simulink model "three"  (R2014b)
settings: Solver=ode23tb  StartTime=0.0  StopTime=0.1  MaxStep=.0001  MinStep=0.00001  RelTol=1e-3
libraries: powerlib x120, simulink x60, powerlib_meascontrol x1
(part 2 of 2)

== system three/R/R/LOOKUP TABLE/If Action Subsystem1 ==
  In1 : Inport
  Action Port : ActionPort  ActionType=case
  Out1 : Outport
  wires:
  In1/1 -> Out1/1

== system three/R/R/LOOKUP TABLE/If Action Subsystem10 ==
  In1 : Inport
  Action Port : ActionPort  ActionType=case
  Out1 : Outport
  wires:
  In1/1 -> Out1/1

== system three/R/R/LOOKUP TABLE/If Action Subsystem2 ==
  In1 : Inport
  Action Port : ActionPort  ActionType=case
  Out1 : Outport
  wires:
  In1/1 -> Out1/1

== system three/R/R/LOOKUP TABLE/If Action Subsystem3 ==
  In1 : Inport
  Action Port : ActionPort  ActionType=case
  Out1 : Outport
  wires:
  In1/1 -> Out1/1

== system three/R/R/LOOKUP TABLE/If Action Subsystem4 ==
  In1 : Inport
  Action Port : ActionPort  ActionType=case
  Out1 : Outport
  wires:
  In1/1 -> Out1/1

== system three/R/R/LOOKUP TABLE/If Action Subsystem5 ==
  In1 : Inport
  Action Port : ActionPort  ActionType=case
  Out1 : Outport
  wires:
  In1/1 -> Out1/1

== system three/R/R/LOOKUP TABLE/If Action Subsystem6 ==
  In1 : Inport
  Action Port : ActionPort  ActionType=case
  Out1 : Outport
  wires:
  In1/1 -> Out1/1

== system three/R/R/LOOKUP TABLE/If Action Subsystem7 ==
  In1 : Inport
  Action Port : ActionPort  ActionType=case
  Out1 : Outport
  wires:
  In1/1 -> Out1/1

== system three/R/R/LOOKUP TABLE/If Action Subsystem8 ==
  In1 : Inport
  Action Port : ActionPort  ActionType=case
  Out1 : Outport
  wires:
  In1/1 -> Out1/1

== system three/R/R/LOOKUP TABLE/If Action Subsystem9 ==
  In1 : Inport
  Action Port : ActionPort  ActionType=case
  Out1 : Outport
  wires:
  In1/1 -> Out1/1

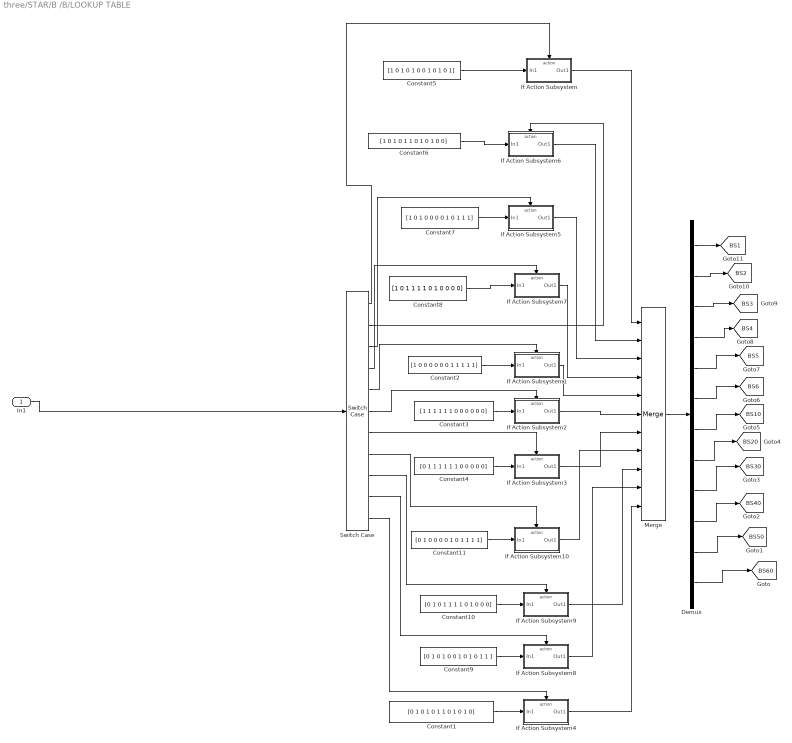
== system three/STAR/B /B/LOOKUP TABLE ==
  In1 : Inport
  Constant1 : Constant  Value=[0 1 0 1 0 1 1 0 1 0 1 0]
  Constant10 : Constant  Value=[0 1 0 1 1 1 1 0 1 0 0 0]
  Constant11 : Constant  Value=[0 1 0 0 0 0 1 0 1 1 1 1]
  Constant2 : Constant  Value=[1 0 0 0 0 0 0 1 1 1 1 1]
  Constant3 : Constant  Value=[1 1 1 1 1 1 0 0 0 0 0 0]
  Constant4 : Constant  Value=[0 1 1 1 1 1 1 0 0 0 0 0]
  Constant5 : Constant  Value=[1 0 1 0 1 0 0 1 0 1 0 1]
  Constant6 : Constant  Value=[1 0 1 0 1 1 0 1 0 1 0 0]
  Constant7 : Constant  Value=[1 0 1 0 0 0 0 1 0 1 1 1]
  Constant8 : Constant  Value=[1 0 1 1 1 1 0 1 0 0 0 0]
  Constant9 : Constant  Value=[0 1 0 1 0 0 1 0 1 0 1 1 ]
  Demux : Demux  Outputs=12
  If Action Subsystem : Subsystem  TreatAsAtomicUnit=on
  If Action Subsystem1 : Subsystem  TreatAsAtomicUnit=on
  If Action Subsystem10 : Subsystem  TreatAsAtomicUnit=on
  If Action Subsystem2 : Subsystem  TreatAsAtomicUnit=on
  If Action Subsystem3 : Subsystem  TreatAsAtomicUnit=on
  If Action Subsystem4 : Subsystem  TreatAsAtomicUnit=on
  If Action Subsystem5 : Subsystem  TreatAsAtomicUnit=on
  If Action Subsystem6 : Subsystem  TreatAsAtomicUnit=on
  If Action Subsystem7 : Subsystem  TreatAsAtomicUnit=on
  If Action Subsystem8 : Subsystem  TreatAsAtomicUnit=on
  If Action Subsystem9 : Subsystem  TreatAsAtomicUnit=on
  Merge : Merge  Inputs=11
  Switch Case : SwitchCase  CaseConditions={-5 -4 -3 -2 -1 0 1 2 3 4 5}  ShowDefaultCase=off
  tag scope: BS10=global, BS1=global, BS20=global, BS2=global, BS30=global, BS3=global, BS40=global, BS4=global, BS50=global, BS5=global, BS60=global, BS6=global
  wires:
  Merge/1 -> Demux/1
  If Action Subsystem/1(Out1) -> Merge/1
  Constant4/1 -> If Action Subsystem3/1(In1)
  Constant3/1 -> If Action Subsystem2/1(In1)
  Constant2/1 -> If Action Subsystem1/1(In1)
  Switch Case/6 -> If Action Subsystem2/Action
  If Action Subsystem6/1(Out1) -> Merge/2
  If Action Subsystem5/1(Out1) -> Merge/3
  If Action Subsystem7/1(Out1) -> Merge/4
  If Action Subsystem1/1(Out1) -> Merge/5
  If Action Subsystem2/1(Out1) -> Merge/6
  If Action Subsystem3/1(Out1) -> Merge/7
  Constant9/1 -> If Action Subsystem8/1(In1)
  Constant10/1 -> If Action Subsystem9/1(In1)
  Constant11/1 -> If Action Subsystem10/1(In1)
  Switch Case/11 -> If Action Subsystem4/Action
  If Action Subsystem4/1(Out1) -> Merge/11
  Switch Case/10 -> If Action Subsystem8/Action
  Switch Case/9 -> If Action Subsystem9/Action
  Switch Case/8 -> If Action Subsystem10/Action
  Switch Case/7 -> If Action Subsystem3/Action
  Switch Case/5 -> If Action Subsystem1/Action
  Switch Case/4 -> If Action Subsystem7/Action
  Switch Case/3 -> If Action Subsystem5/Action
  Switch Case/2 -> If Action Subsystem6/Action
  Switch Case/1 -> If Action Subsystem/Action
  Constant6/1 -> If Action Subsystem6/1(In1)
  Constant7/1 -> If Action Subsystem5/1(In1)
  Constant8/1 -> If Action Subsystem7/1(In1)
  If Action Subsystem10/1(Out1) -> Merge/8
  If Action Subsystem9/1(Out1) -> Merge/9
  If Action Subsystem8/1(Out1) -> Merge/10
  Constant1/1 -> If Action Subsystem4/1(In1)
  Constant5/1 -> If Action Subsystem/1(In1)
  In1/1 -> Switch Case/1
  Demux/1 -> [BS1]
  Demux/2 -> [BS2]
  Demux/3 -> [BS3]
  Demux/4 -> [BS4]
  Demux/6 -> [BS6]
  Demux/5 -> [BS5]
  Demux/7 -> [BS10]
  Demux/8 -> [BS20]
  Demux/11 -> [BS50]
  Demux/10 -> [BS40]
  Demux/9 -> [BS30]
  Demux/12 -> [BS60]

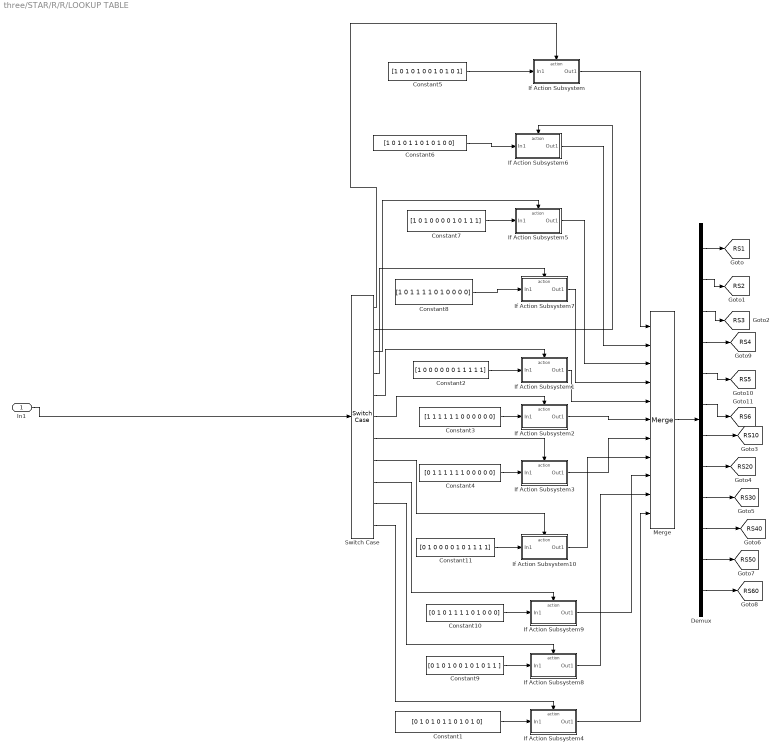
== system three/STAR/R/R/LOOKUP TABLE ==
  In1 : Inport
  Constant1 : Constant  Value=[0 1 0 1 0 1 1 0 1 0 1 0]
  Constant10 : Constant  Value=[0 1 0 1 1 1 1 0 1 0 0 0]
  Constant11 : Constant  Value=[0 1 0 0 0 0 1 0 1 1 1 1]
  Constant2 : Constant  Value=[1 0 0 0 0 0 0 1 1 1 1 1]
  Constant3 : Constant  Value=[1 1 1 1 1 1 0 0 0 0 0 0]
  Constant4 : Constant  Value=[0 1 1 1 1 1 1 0 0 0 0 0]
  Constant5 : Constant  Value=[1 0 1 0 1 0 0 1 0 1 0 1]
  Constant6 : Constant  Value=[1 0 1 0 1 1 0 1 0 1 0 0]
  Constant7 : Constant  Value=[1 0 1 0 0 0 0 1 0 1 1 1]
  Constant8 : Constant  Value=[1 0 1 1 1 1 0 1 0 0 0 0]
  Constant9 : Constant  Value=[0 1 0 1 0 0 1 0 1 0 1 1 ]
  Demux : Demux  Outputs=12
  If Action Subsystem : Subsystem  TreatAsAtomicUnit=on
  If Action Subsystem1 : Subsystem  TreatAsAtomicUnit=on
  If Action Subsystem10 : Subsystem  TreatAsAtomicUnit=on
  If Action Subsystem2 : Subsystem  TreatAsAtomicUnit=on
  If Action Subsystem3 : Subsystem  TreatAsAtomicUnit=on
  If Action Subsystem4 : Subsystem  TreatAsAtomicUnit=on
  If Action Subsystem5 : Subsystem  TreatAsAtomicUnit=on
  If Action Subsystem6 : Subsystem  TreatAsAtomicUnit=on
  If Action Subsystem7 : Subsystem  TreatAsAtomicUnit=on
  If Action Subsystem8 : Subsystem  TreatAsAtomicUnit=on
  If Action Subsystem9 : Subsystem  TreatAsAtomicUnit=on
  Merge : Merge  Inputs=11
  Switch Case : SwitchCase  CaseConditions={-5 -4 -3 -2 -1 0 1 2 3 4 5}  ShowDefaultCase=off
  tag scope: RS10=global, RS1=global, RS20=global, RS2=global, RS30=global, RS3=global, RS40=global, RS4=global, RS50=global, RS5=global, RS60=global, RS6=global
  wires:
  Merge/1 -> Demux/1
  If Action Subsystem/1(Out1) -> Merge/1
  Constant4/1 -> If Action Subsystem3/1(In1)
  Constant3/1 -> If Action Subsystem2/1(In1)
  Constant2/1 -> If Action Subsystem1/1(In1)
  Switch Case/6 -> If Action Subsystem2/Action
  If Action Subsystem6/1(Out1) -> Merge/2
  If Action Subsystem5/1(Out1) -> Merge/3
  If Action Subsystem7/1(Out1) -> Merge/4
  If Action Subsystem1/1(Out1) -> Merge/5
  If Action Subsystem2/1(Out1) -> Merge/6
  If Action Subsystem3/1(Out1) -> Merge/7
  Constant9/1 -> If Action Subsystem8/1(In1)
  Constant10/1 -> If Action Subsystem9/1(In1)
  Constant11/1 -> If Action Subsystem10/1(In1)
  Switch Case/11 -> If Action Subsystem4/Action
  If Action Subsystem4/1(Out1) -> Merge/11
  Switch Case/10 -> If Action Subsystem8/Action
  Switch Case/9 -> If Action Subsystem9/Action
  Switch Case/8 -> If Action Subsystem10/Action
  Switch Case/7 -> If Action Subsystem3/Action
  Switch Case/5 -> If Action Subsystem1/Action
  Switch Case/4 -> If Action Subsystem7/Action
  Switch Case/3 -> If Action Subsystem5/Action
  Switch Case/2 -> If Action Subsystem6/Action
  Switch Case/1 -> If Action Subsystem/Action
  Constant6/1 -> If Action Subsystem6/1(In1)
  Constant7/1 -> If Action Subsystem5/1(In1)
  Constant8/1 -> If Action Subsystem7/1(In1)
  If Action Subsystem10/1(Out1) -> Merge/8
  If Action Subsystem9/1(Out1) -> Merge/9
  If Action Subsystem8/1(Out1) -> Merge/10
  Demux/3 -> [RS3]
  Demux/2 -> [RS2]
  Demux/1 -> [RS1]
  Demux/7 -> [RS10]
  Demux/8 -> [RS20]
  Demux/9 -> [RS30]
  Demux/10 -> [RS40]
  Demux/11 -> [RS50]
  Demux/12 -> [RS60]
  Demux/6 -> [RS6]
  Demux/5 -> [RS5]
  Demux/4 -> [RS4]
  Constant1/1 -> If Action Subsystem4/1(In1)
  Constant5/1 -> If Action Subsystem/1(In1)
  In1/1 -> Switch Case/1

== system three/STAR/Y/B/LOOKUP TABLE ==
  In1 : Inport
  Constant1 : Constant  Value=[0 1 0 1 0 1 1 0 1 0 1 0]
  Constant10 : Constant  Value=[0 1 0 1 1 1 1 0 1 0 0 0]
  Constant11 : Constant  Value=[0 1 0 0 0 0 1 0 1 1 1 1]
  Constant2 : Constant  Value=[1 0 0 0 0 0 0 1 1 1 1 1]
  Constant3 : Constant  Value=[1 1 1 1 1 1 0 0 0 0 0 0]
  Constant4 : Constant  Value=[0 1 1 1 1 1 1 0 0 0 0 0]
  Constant5 : Constant  Value=[1 0 1 0 1 0 0 1 0 1 0 1]
  Constant6 : Constant  Value=[1 0 1 0 1 1 0 1 0 1 0 0]
  Constant7 : Constant  Value=[1 0 1 0 0 0 0 1 0 1 1 1]
  Constant8 : Constant  Value=[1 0 1 1 1 1 0 1 0 0 0 0]
  Constant9 : Constant  Value=[0 1 0 1 0 0 1 0 1 0 1 1 ]
  Demux : Demux  Outputs=12
  If Action Subsystem : Subsystem  TreatAsAtomicUnit=on
  If Action Subsystem1 : Subsystem  TreatAsAtomicUnit=on
  If Action Subsystem10 : Subsystem  TreatAsAtomicUnit=on
  If Action Subsystem2 : Subsystem  TreatAsAtomicUnit=on
  If Action Subsystem3 : Subsystem  TreatAsAtomicUnit=on
  If Action Subsystem4 : Subsystem  TreatAsAtomicUnit=on
  If Action Subsystem5 : Subsystem  TreatAsAtomicUnit=on
  If Action Subsystem6 : Subsystem  TreatAsAtomicUnit=on
  If Action Subsystem7 : Subsystem  TreatAsAtomicUnit=on
  If Action Subsystem8 : Subsystem  TreatAsAtomicUnit=on
  If Action Subsystem9 : Subsystem  TreatAsAtomicUnit=on
  Merge : Merge  Inputs=11
  Switch Case : SwitchCase  CaseConditions={-5 -4 -3 -2 -1 0 1 2 3 4 5}  ShowDefaultCase=off
  tag scope: YS10=global, YS20=global, YS2=global, YS30=global, YS3=global, YS40=global, YS4=global, YS50=global, YS5=global, YS60=global, YS6=global
  wires:
  In1/1 -> Switch Case/1
  Constant5/1 -> If Action Subsystem/1(In1)
  Constant1/1 -> If Action Subsystem4/1(In1)
  If Action Subsystem8/1(Out1) -> Merge/10
  If Action Subsystem9/1(Out1) -> Merge/9
  If Action Subsystem10/1(Out1) -> Merge/8
  Constant8/1 -> If Action Subsystem7/1(In1)
  Constant7/1 -> If Action Subsystem5/1(In1)
  Constant6/1 -> If Action Subsystem6/1(In1)
  Switch Case/1 -> If Action Subsystem/Action
  Switch Case/2 -> If Action Subsystem6/Action
  Switch Case/3 -> If Action Subsystem5/Action
  Switch Case/4 -> If Action Subsystem7/Action
  Switch Case/5 -> If Action Subsystem1/Action
  Switch Case/7 -> If Action Subsystem3/Action
  Switch Case/8 -> If Action Subsystem10/Action
  Switch Case/9 -> If Action Subsystem9/Action
  Switch Case/10 -> If Action Subsystem8/Action
  If Action Subsystem4/1(Out1) -> Merge/11
  Switch Case/11 -> If Action Subsystem4/Action
  Constant11/1 -> If Action Subsystem10/1(In1)
  Constant10/1 -> If Action Subsystem9/1(In1)
  Constant9/1 -> If Action Subsystem8/1(In1)
  If Action Subsystem3/1(Out1) -> Merge/7
  If Action Subsystem2/1(Out1) -> Merge/6
  If Action Subsystem1/1(Out1) -> Merge/5
  If Action Subsystem7/1(Out1) -> Merge/4
  If Action Subsystem5/1(Out1) -> Merge/3
  If Action Subsystem6/1(Out1) -> Merge/2
  Switch Case/6 -> If Action Subsystem2/Action
  Constant2/1 -> If Action Subsystem1/1(In1)
  Constant3/1 -> If Action Subsystem2/1(In1)
  Constant4/1 -> If Action Subsystem3/1(In1)
  If Action Subsystem/1(Out1) -> Merge/1
  Merge/1 -> Demux/1
  Demux/1 -> [YS1]
  Demux/3 -> [YS3]
  Demux/2 -> [YS2]
  Demux/4 -> [YS4]
  Demux/5 -> [YS5]
  Demux/6 -> [YS6]
  Demux/7 -> [YS10]
  Demux/8 -> [YS20]
  Demux/9 -> [YS30]
  Demux/10 -> [YS40]
  Demux/11 -> [YS50]
  Demux/12 -> [YS60]

== system three/Y/Y/LOOKUP TABLE/If Action Subsystem ==
  In1 : Inport
  Action Port : ActionPort  ActionType=case
  Out1 : Outport
  wires:
  In1/1 -> Out1/1

== system three/Y/Y/LOOKUP TABLE/If Action Subsystem1 ==
  In1 : Inport
  Action Port : ActionPort  ActionType=case
  Out1 : Outport
  wires:
  In1/1 -> Out1/1

== system three/Y/Y/LOOKUP TABLE/If Action Subsystem10 ==
  In1 : Inport
  Action Port : ActionPort  ActionType=case
  Out1 : Outport
  wires:
  In1/1 -> Out1/1

== system three/Y/Y/LOOKUP TABLE/If Action Subsystem2 ==
  In1 : Inport
  Action Port : ActionPort  ActionType=case
  Out1 : Outport
  wires:
  In1/1 -> Out1/1

== system three/Y/Y/LOOKUP TABLE/If Action Subsystem3 ==
  In1 : Inport
  Action Port : ActionPort  ActionType=case
  Out1 : Outport
  wires:
  In1/1 -> Out1/1

== system three/Y/Y/LOOKUP TABLE/If Action Subsystem4 ==
  In1 : Inport
  Action Port : ActionPort  ActionType=case
  Out1 : Outport
  wires:
  In1/1 -> Out1/1

== system three/Y/Y/LOOKUP TABLE/If Action Subsystem5 ==
  In1 : Inport
  Action Port : ActionPort  ActionType=case
  Out1 : Outport
  wires:
  In1/1 -> Out1/1

== system three/Y/Y/LOOKUP TABLE/If Action Subsystem6 ==
  In1 : Inport
  Action Port : ActionPort  ActionType=case
  Out1 : Outport
  wires:
  In1/1 -> Out1/1

== system three/Y/Y/LOOKUP TABLE/If Action Subsystem7 ==
  In1 : Inport
  Action Port : ActionPort  ActionType=case
  Out1 : Outport
  wires:
  In1/1 -> Out1/1

== system three/Y/Y/LOOKUP TABLE/If Action Subsystem8 ==
  In1 : Inport
  Action Port : ActionPort  ActionType=case
  Out1 : Outport
  wires:
  In1/1 -> Out1/1

== system three/Y/Y/LOOKUP TABLE/If Action Subsystem9 ==
  In1 : Inport
  Action Port : ActionPort  ActionType=case
  Out1 : Outport
  wires:
  In1/1 -> Out1/1

== system three/STAR/B /B/LOOKUP TABLE/If Action Subsystem ==
  In1 : Inport
  Action Port : ActionPort
  Out1 : Outport
  wires:
  In1/1 -> Out1/1

== system three/STAR/B /B/LOOKUP TABLE/If Action Subsystem1 ==
  In1 : Inport
  Action Port : ActionPort
  Out1 : Outport
  wires:
  In1/1 -> Out1/1

== system three/STAR/B /B/LOOKUP TABLE/If Action Subsystem10 ==
  In1 : Inport
  Action Port : ActionPort
  Out1 : Outport
  wires:
  In1/1 -> Out1/1

== system three/STAR/B /B/LOOKUP TABLE/If Action Subsystem2 ==
  In1 : Inport
  Action Port : ActionPort
  Out1 : Outport
  wires:
  In1/1 -> Out1/1

== system three/STAR/B /B/LOOKUP TABLE/If Action Subsystem3 ==
  In1 : Inport
  Action Port : ActionPort
  Out1 : Outport
  wires:
  In1/1 -> Out1/1

== system three/STAR/B /B/LOOKUP TABLE/If Action Subsystem4 ==
  In1 : Inport
  Action Port : ActionPort
  Out1 : Outport
  wires:
  In1/1 -> Out1/1

== system three/STAR/B /B/LOOKUP TABLE/If Action Subsystem5 ==
  In1 : Inport
  Action Port : ActionPort
  Out1 : Outport
  wires:
  In1/1 -> Out1/1

== system three/STAR/B /B/LOOKUP TABLE/If Action Subsystem6 ==
  In1 : Inport
  Action Port : ActionPort
  Out1 : Outport
  wires:
  In1/1 -> Out1/1

== system three/STAR/B /B/LOOKUP TABLE/If Action Subsystem7 ==
  In1 : Inport
  Action Port : ActionPort
  Out1 : Outport
  wires:
  In1/1 -> Out1/1

== system three/STAR/B /B/LOOKUP TABLE/If Action Subsystem8 ==
  In1 : Inport
  Action Port : ActionPort
  Out1 : Outport
  wires:
  In1/1 -> Out1/1

== system three/STAR/B /B/LOOKUP TABLE/If Action Subsystem9 ==
  In1 : Inport
  Action Port : ActionPort
  Out1 : Outport
  wires:
  In1/1 -> Out1/1

== system three/STAR/R/R/LOOKUP TABLE/If Action Subsystem ==
  In1 : Inport
  Action Port : ActionPort
  Out1 : Outport
  wires:
  In1/1 -> Out1/1

== system three/STAR/R/R/LOOKUP TABLE/If Action Subsystem1 ==
  In1 : Inport
  Action Port : ActionPort
  Out1 : Outport
  wires:
  In1/1 -> Out1/1

== system three/STAR/R/R/LOOKUP TABLE/If Action Subsystem10 ==
  In1 : Inport
  Action Port : ActionPort
  Out1 : Outport
  wires:
  In1/1 -> Out1/1

== system three/STAR/R/R/LOOKUP TABLE/If Action Subsystem2 ==
  In1 : Inport
  Action Port : ActionPort
  Out1 : Outport
  wires:
  In1/1 -> Out1/1

== system three/STAR/R/R/LOOKUP TABLE/If Action Subsystem3 ==
  In1 : Inport
  Action Port : ActionPort
  Out1 : Outport
  wires:
  In1/1 -> Out1/1

== system three/STAR/R/R/LOOKUP TABLE/If Action Subsystem4 ==
  In1 : Inport
  Action Port : ActionPort
  Out1 : Outport
  wires:
  In1/1 -> Out1/1

== system three/STAR/R/R/LOOKUP TABLE/If Action Subsystem5 ==
  In1 : Inport
  Action Port : ActionPort
  Out1 : Outport
  wires:
  In1/1 -> Out1/1

== system three/STAR/R/R/LOOKUP TABLE/If Action Subsystem6 ==
  In1 : Inport
  Action Port : ActionPort
  Out1 : Outport
  wires:
  In1/1 -> Out1/1

== system three/STAR/R/R/LOOKUP TABLE/If Action Subsystem7 ==
  In1 : Inport
  Action Port : ActionPort
  Out1 : Outport
  wires:
  In1/1 -> Out1/1

== system three/STAR/R/R/LOOKUP TABLE/If Action Subsystem8 ==
  In1 : Inport
  Action Port : ActionPort
  Out1 : Outport
  wires:
  In1/1 -> Out1/1

== system three/STAR/R/R/LOOKUP TABLE/If Action Subsystem9 ==
  In1 : Inport
  Action Port : ActionPort
  Out1 : Outport
  wires:
  In1/1 -> Out1/1

== system three/STAR/Y/B/LOOKUP TABLE/If Action Subsystem ==
  In1 : Inport
  Action Port : ActionPort
  Out1 : Outport
  wires:
  In1/1 -> Out1/1

== system three/STAR/Y/B/LOOKUP TABLE/If Action Subsystem1 ==
  In1 : Inport
  Action Port : ActionPort
  Out1 : Outport
  wires:
  In1/1 -> Out1/1

== system three/STAR/Y/B/LOOKUP TABLE/If Action Subsystem10 ==
  In1 : Inport
  Action Port : ActionPort
  Out1 : Outport
  wires:
  In1/1 -> Out1/1

== system three/STAR/Y/B/LOOKUP TABLE/If Action Subsystem2 ==
  In1 : Inport
  Action Port : ActionPort
  Out1 : Outport
  wires:
  In1/1 -> Out1/1

== system three/STAR/Y/B/LOOKUP TABLE/If Action Subsystem3 ==
  In1 : Inport
  Action Port : ActionPort
  Out1 : Outport
  wires:
  In1/1 -> Out1/1

== system three/STAR/Y/B/LOOKUP TABLE/If Action Subsystem4 ==
  In1 : Inport
  Action Port : ActionPort
  Out1 : Outport
  wires:
  In1/1 -> Out1/1

== system three/STAR/Y/B/LOOKUP TABLE/If Action Subsystem5 ==
  In1 : Inport
  Action Port : ActionPort
  Out1 : Outport
  wires:
  In1/1 -> Out1/1

== system three/STAR/Y/B/LOOKUP TABLE/If Action Subsystem6 ==
  In1 : Inport
  Action Port : ActionPort
  Out1 : Outport
  wires:
  In1/1 -> Out1/1

== system three/STAR/Y/B/LOOKUP TABLE/If Action Subsystem7 ==
  In1 : Inport
  Action Port : ActionPort
  Out1 : Outport
  wires:
  In1/1 -> Out1/1

== system three/STAR/Y/B/LOOKUP TABLE/If Action Subsystem8 ==
  In1 : Inport
  Action Port : ActionPort
  Out1 : Outport
  wires:
  In1/1 -> Out1/1

== system three/STAR/Y/B/LOOKUP TABLE/If Action Subsystem9 ==
  In1 : Inport
  Action Port : ActionPort
  Out1 : Outport
  wires:
  In1/1 -> Out1/1
